simulink model "multifusion2"  (R2023b)
settings: Solver=VariableStepAuto  StartTime=0.0  StopTime=10.0  RelTol=1e-3
settings Model: Creator=anruk  LastModifiedBy=anruk

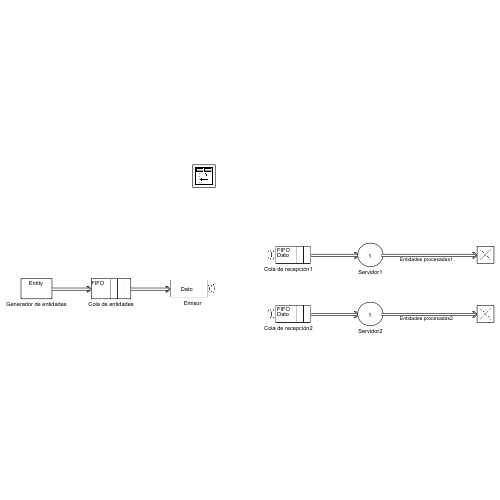
[thumbnail: Simulink's stored preview of the top-level diagram]
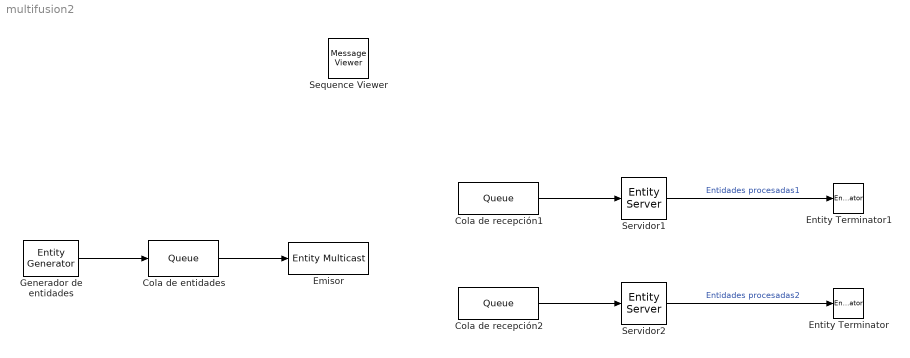
== system multifusion2 ==
  Cola de entidades : Queue  InputPortMessageModes=m  OutputPortMessageModes=m
  Cola de recepción1 : Queue  OutputPortMessageModes=m  EntityArrivalSource=Multicast  MulticastTag=Dato
  Cola de recepción2 : Queue  OutputPortMessageModes=m  EntityArrivalSource=Multicast  MulticastTag=Dato
  Emisor : EntityMulticast  Tag=Dato  InputPortMessageModes=m  MulticastTag=Dato
  Entity Terminator : EntityTerminator  InputPortMessageModes=m
  Entity Terminator1 : EntityTerminator  InputPortMessageModes=m
  Generador de entidades : EntityGenerator  OutputPortMessageModes=m  TimeSource=MATLAB action  EntityType=Structured  EntityTypeName=Entity
  Sequence Viewer : MessageViewer  History=1000  SavedRootId=#
  Servidor1 : EntityServer  InputPortMessageModes=m  OutputPortMessageModes=m  Capacity=1  ServiceTimeValue=2
  Servidor2 : EntityServer  InputPortMessageModes=m  OutputPortMessageModes=m  Capacity=1  ServiceTimeValue=2
  wires:
  Cola de recepción2/1 -> Servidor2/1
  Generador de entidades/1 -> Cola de entidades/1
  Cola de entidades/1 -> Emisor/1
  Servidor2/1 -> Entity Terminator/1  "Entidades procesadas2"
  Servidor1/1 -> Entity Terminator1/1  "Entidades procesadas1"
  Cola de recepción1/1 -> Servidor1/1
